simulink library "FlattenAircraftEstimateBus"  (R2018b)
settings: Solver=VariableStepAuto  StartTime=0.0  StopTime=10.0  RelTol=1e-3
settings Model: Creator=BI28030  LastModifiedBy=BI28030

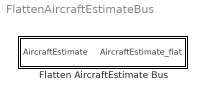
== system FlattenAircraftEstimateBus ==
  Flatten AircraftEstimate Bus : Subsystem

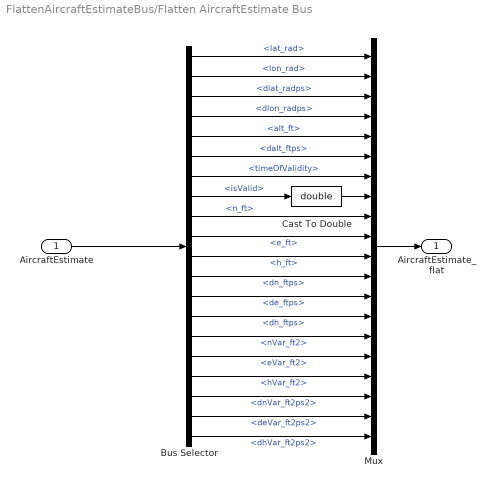
== system FlattenAircraftEstimateBus/Flatten AircraftEstimate Bus ==
  AircraftEstimate : Inport
  Bus Selector : BusSelector  OutputSignals=latLonAltEst.lat_rad,latLonAltEst.lon_rad,latLonAltEst.dlat_radps,latLonAltEst.dlon_radps,latLonAltEst.alt_ft,latLonAltEst.dalt_ftps,timeOfValidity,isValid,enuStateEstimate.n_ft,enuStateEstimate.e_ft,enuStateEstimate.h_ft,enuStateEstimate.dn_ftps,enuStateEstimate.de_ftps,enuStateEstimate.dh_ftps,covEstimate.nVar_ft2,covEstimate.eVar_ft2,covEstimate.hVar_ft2,covEstimate.dnVar_ft2ps2,covEstimate.deVar_ft2ps2,covEstimate.dhVar_ft2ps2
  Cast To Double : DataTypeConversion  OutDataTypeStr=double
  Mux : Mux  Inputs=20
  AircraftEstimate_flat : Outport
  wires:
  AircraftEstimate/1 -> Bus Selector/1
  Bus Selector/1 -> Mux/1  "<lat_rad>"
  Bus Selector/2 -> Mux/2  "<lon_rad>"
  Bus Selector/3 -> Mux/3  "<dlat_radps>"
  Bus Selector/4 -> Mux/4  "<dlon_radps>"
  Bus Selector/5 -> Mux/5  "<alt_ft>"
  Bus Selector/6 -> Mux/6  "<dalt_ftps>"
  Bus Selector/7 -> Mux/7  "<timeOfValidity>"
  Bus Selector/8 -> Cast To Double/1  "<isValid>"
  Bus Selector/9 -> Mux/9  "<n_ft>"
  Bus Selector/10 -> Mux/10  "<e_ft>"
  Bus Selector/11 -> Mux/11  "<h_ft>"
  Bus Selector/12 -> Mux/12  "<dn_ftps>"
  Bus Selector/13 -> Mux/13  "<de_ftps>"
  Bus Selector/14 -> Mux/14  "<dh_ftps>"
  Bus Selector/15 -> Mux/15  "<nVar_ft2>"
  Bus Selector/16 -> Mux/16  "<eVar_ft2>"
  Bus Selector/17 -> Mux/17  "<hVar_ft2>"
  Bus Selector/18 -> Mux/18  "<dnVar_ft2ps2>"
  Bus Selector/19 -> Mux/19  "<deVar_ft2ps2>"
  Bus Selector/20 -> Mux/20  "<dhVar_ft2ps2>"
  Mux/1 -> AircraftEstimate_flat/1
  Cast To Double/1 -> Mux/8
